simulink model "full_block_trim"  (R2014a)
settings: Solver=ode45  StartTime=0.0  StopTime=500.0  RelTol=1e-3
values from neighbouring files (symbols this model uses):
  alpha_dot = 0    [init_coeff_Cessna.m]
  b = 10.911    [init_coeff_Cessna.m]
  c_bar = 1.493    [init_coeff_Cessna.m]
  c_l_beta = -0.089    [init_coeff_Cessna.m]
  c_l_delta_a = -0.09    [init_coeff_Cessna.m]
  c_l_delta_r = 0.0147    [init_coeff_Cessna.m]
  c_l_p = -0.47    [init_coeff_Cessna.m]
  c_l_r = 0.096    [init_coeff_Cessna.m]
  cd0 = 0.036    [init_coeff_Cessna.m]
  cd_alpha = 0.13    [init_coeff_Cessna.m]
  cd_beta = 0.17    [init_coeff_Cessna.m]
  cd_delta_e = 0.06    [init_coeff_Cessna.m]
  cl0 = 0.25    [init_coeff_Cessna.m]
  cl_alpha = 4.47    [init_coeff_Cessna.m]
  cl_delta_e = 0.3476    [init_coeff_Cessna.m]
  cl_q = 3.9    [init_coeff_Cessna.m]
  cm0 = -0.02    [init_coeff_Cessna.m]
  cm_alpha = -1.8    [init_coeff_Cessna.m]
  cm_alpha_dot = 0.0    (= 0)    [init_coeff_Cessna.m]
  cm_delta_e = -1.28    [init_coeff_Cessna.m]
  cn_beta = 0.065    [init_coeff_Cessna.m]
  cn_delta_a = -0.0053    [init_coeff_Cessna.m]
  cn_delta_r = -0.0657    [init_coeff_Cessna.m]
  cn_p = -0.03    [init_coeff_Cessna.m]
  cn_r = -0.99    [init_coeff_Cessna.m]
  cy_beta = -0.31    [init_coeff_Cessna.m]
  cy_delta_a = 0    [init_coeff_Cessna.m]
  cy_p = -0.037    [init_coeff_Cessna.m]
  cy_r = 0.21    [init_coeff_Cessna.m]
  Ixx = 1285.31    [init_coeff_Cessna.m]
  Ixy = 0.0    (= 0)    [init_coeff_Cessna.m]
  Ixz = 0.0    (= 0)    [init_coeff_Cessna.m]
  Iyx = Ixy    (= 0)    [init_coeff_Cessna.m]
  Iyy = 1824.93    [init_coeff_Cessna.m]
  Iyz = 0.0    (= 0)    [init_coeff_Cessna.m]
  Izx = Ixz    (= 0)    [init_coeff_Cessna.m]
  Izy = Iyz    (= 0)    [init_coeff_Cessna.m]
  Izz = 2666.893    [init_coeff_Cessna.m]
  k_drag = 0.0830304    [init_coeff_Cessna.m]
  p_init = 0    [trim_simulate.m]
  phi_init = 0    [trim_simulate.m]
  psi_init = 0    [trim_simulate.m]
  q_init = 0    [trim_simulate.m]
  r_init = 0    [trim_simulate.m]
  S = 16.1651    [init_coeff_Cessna.m]
  theta_init = 0.0105    [trim_simulate.m]
  u_init = 80.00    (= 80)    [trim_simulate.m]
  v_init = 0.00    (= 0)    [trim_simulate.m]
  W = mass*g    (= 10223.948)    [init_coeff_Cessna.m]
  w_init = 0    [trim_simulate.m]
  xe_init = 0    [trim_simulate.m]
  ye_init = 0    [trim_simulate.m]
  ze_init = -200    [trim_simulate.m]
libraries: aerolibobsolete x1, aerolibatmos2 x1, aerolibtransform2 x1, aerolibasang x1
settings Model: Creator=sajith  LastModifiedBy=sajith
settings DataIOCC: SignalLoggingSaveFormat=ModelDataLogs
settings OptimizationCC: ExpressionDepthLimit=2147483647
settings DebuggingCC: UnderspecifiedInitializationDetection=Classic  FcnCallInpInsideContextMsg=UseLocalSettings  StateNameClashWarn=warning
settings SFSimCC: SimParseCustomCode=off
settings GRTTargetCC: CombineOutputUpdateFcns=off  GRTInterface=on

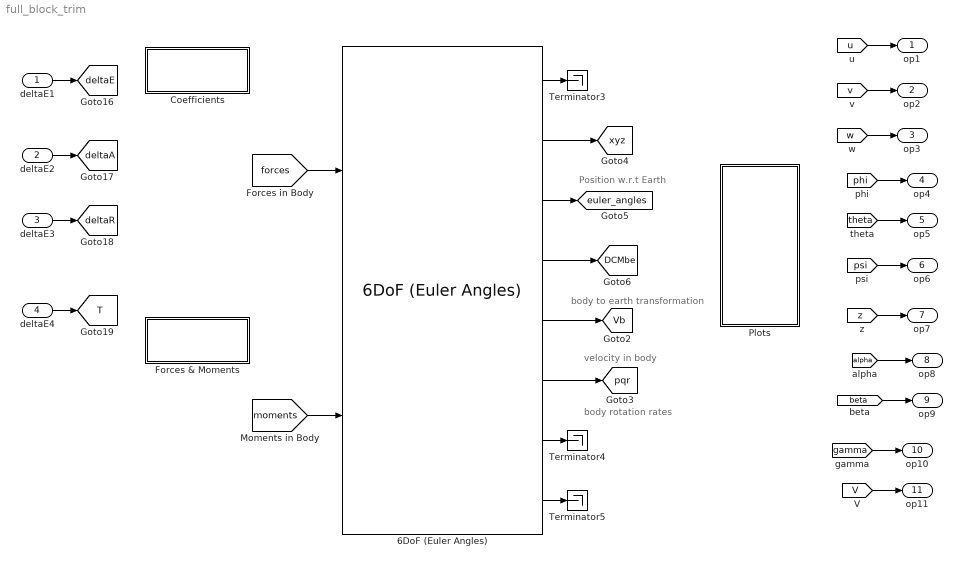
== system full_block_trim ==
  note: velocity in body
  note: body rotation rates
  note: body to earth transformation
  note: Position w.r.t Earth
  deltaE1 : Inport
  deltaE2 : Inport  Port=2
  deltaE3 : Inport  Port=3
  deltaE4 : Inport  Port=4
  6DoF (Euler Angles) : aerolibobsolete/6DoF (Euler Angles)  units=Metric (MKS)  mtype=Fixed  rep=Euler Angles  xme_0=[xe_init ye_init ze_init]  Vm_0=[u_init v_init w_init]  eul_0=[phi_init theta_init psi_init]  pm_0=[p_init q_init r_init]  mass_0=mass  mass_e=0.5  mass_f=2.0  inertia=[Ixx Ixy Ixz;Iyx Iyy Iyz;Izx Izy Izz]  inertia_e=eye(3)  inertia_f=2*eye(3)  k_quat=1.0
  Coefficients : Subsystem
  Forces & Moments : Subsystem
  Plots : Subsystem
  Terminator3 : Terminator
  Terminator4 : Terminator
  Terminator5 : Terminator
  op1 : Outport
  op2 : Outport  Port=2
  op3 : Outport  Port=3
  op4 : Outport  Port=4
  op5 : Outport  Port=5
  op6 : Outport  Port=6
  op7 : Outport  Port=7
  op8 : Outport  Port=8
  op9 : Outport  Port=9
  op10 : Outport  Port=10
  op11 : Outport  Port=11
  tag scope: DCMbe=global, T=global, Vb=global, deltaA=global, deltaE=global, deltaR=global, euler_angles=global, pqr=global, xyz=global
  wires:
  deltaE2/1 -> [deltaA]
  deltaE3/1 -> [deltaR]
  deltaE1/1 -> [deltaE]
  deltaE4/1 -> [T]
  [u] -> op1/1
  [v] -> op2/1
  [w] -> op3/1
  [phi] -> op4/1
  [theta] -> op5/1
  [psi] -> op6/1
  [z] -> op7/1
  [alpha] -> op8/1
  [beta] -> op9/1
  [gamma] -> op10/1
  [V] -> op11/1
  [forces] -> 6DoF (Euler Angles)/1
  [moments] -> 6DoF (Euler Angles)/2
  6DoF (Euler Angles)/2 -> [xyz]
  6DoF (Euler Angles)/3 -> [euler_angles]
  6DoF (Euler Angles)/4 -> [DCMbe]
  6DoF (Euler Angles)/6 -> [pqr]
  6DoF (Euler Angles)/5 -> [Vb]
  6DoF (Euler Angles)/1 -> Terminator3/1
  6DoF (Euler Angles)/7 -> Terminator4/1
  6DoF (Euler Angles)/8 -> Terminator5/1

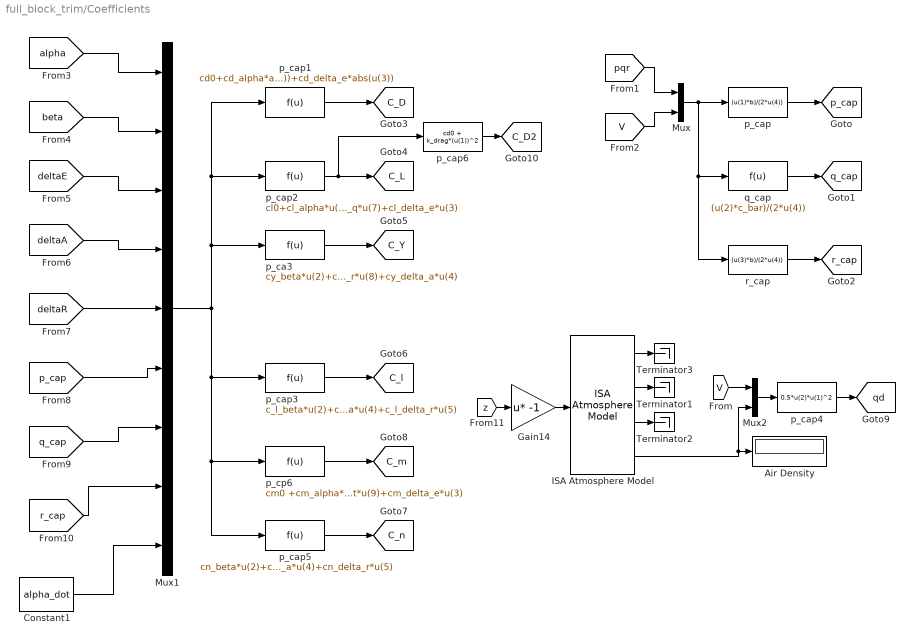
== system full_block_trim/Coefficients ==
  Air Density : Display
  Constant1 : Constant  Value=alpha_dot
  Gain14 : Gain  Gain=-1  Multiplication=Matrix(u*K)
  ISA Atmosphere Model : aerolibatmos2/ISA Atmosphere Model  custom=off  g=9.80665  gamma=1.4  R=287.0531  L=0.0065  h_trop=11000  h_strat=20000  rho0=1.225  P0=101325  T0=288.15  h0=0
  Mux : Mux  Inputs=2
  Mux1 : Mux  Inputs=9
  Mux2 : Mux  Inputs=2
  Terminator1 : Terminator
  Terminator2 : Terminator
  Terminator3 : Terminator
  p_ca3 : Fcn  Expr=cy_beta*u(2)+cy_p*u(6)+cy_r*u(8)+cy_delta_a*u(4)
  p_cap : Fcn  Expr=(u(1)*b)/(2*u(4))
  p_cap1 : Fcn  Expr=cd0+cd_alpha*abs(u(1))+cd_beta*abs(u(2))+cd_delta_e*abs(u(3))
  p_cap2 : Fcn  Expr=cl0+cl_alpha*u(1)+cl_q*u(7)+cl_delta_e*u(3)
  p_cap3 : Fcn  Expr=c_l_beta*u(2)+c_l_p*u(6)+c_l_r*u(8)+c_l_delta_a*u(4)+c_l_delta_r*u(5)
  p_cap4 : Fcn  Expr=0.5*u(2)*u(1)^2
  p_cap5 : Fcn  Expr=cn_beta*u(2)+cn_p*u(6)+cn_r*u(8)+cn_delta_a*u(4)+cn_delta_r*u(5)
  p_cap6 : Fcn  Expr=cd0 + k_drag*(u(1))^2
  p_cp6 : Fcn  Expr=cm0 +cm_alpha*u(1)+cm_alpha_dot*u(9)+cm_delta_e*u(3)
  q_cap : Fcn  Expr=(u(2)*c_bar)/(2*u(4))
  r_cap : Fcn  Expr=(u(3)*b)/(2*u(4))
  tag scope: C_D2=global, C_D=global, C_L=global, C_Y=global, C_l=global, C_m=global, C_n=global, p_cap=global, q_cap=global, qd=global, r_cap=global
  wires:
  [pqr] -> Mux/1
  [V] -> Mux/2
  Mux/1 -> p_cap/1, q_cap/1, r_cap/1
  p_cap/1 -> [p_cap]
  q_cap/1 -> [q_cap]
  r_cap/1 -> [r_cap]
  [alpha] -> Mux1/1
  [beta] -> Mux1/2
  [deltaE] -> Mux1/3
  [deltaA] -> Mux1/4
  [deltaR] -> Mux1/5
  [p_cap] -> Mux1/6
  [q_cap] -> Mux1/7
  [r_cap] -> Mux1/8
  Constant1/1 -> Mux1/9
  Mux1/1 -> p_cap1/1, p_cap2/1, p_ca3/1, p_cap3/1, p_cp6/1, p_cap5/1
  p_cap1/1 -> [C_D]
  p_ca3/1 -> [C_Y]
  p_cap3/1 -> [C_l]
  p_cap5/1 -> [C_n]
  p_cp6/1 -> [C_m]
  [V] -> Mux2/1
  Mux2/1 -> p_cap4/1
  p_cap4/1 -> [qd]
  ISA Atmosphere Model/4 -> Air Density/1, Mux2/2
  Gain14/1 -> ISA Atmosphere Model/1
  [z] -> Gain14/1
  ISA Atmosphere Model/1 -> Terminator3/1
  ISA Atmosphere Model/2 -> Terminator1/1
  ISA Atmosphere Model/3 -> Terminator2/1
  p_cap2/1 -> p_cap6/1, [C_L]
  p_cap6/1 -> [C_D2]

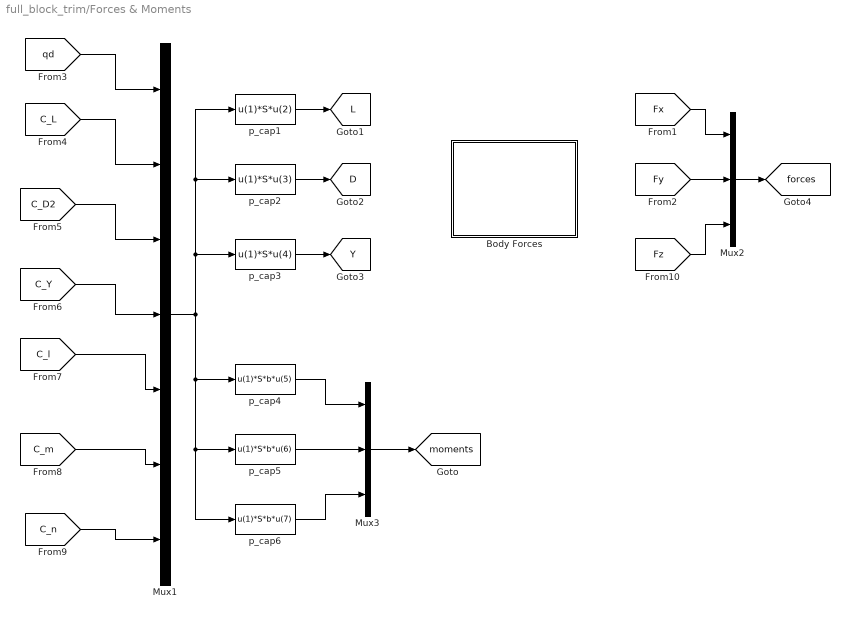
== system full_block_trim/Forces & Moments ==
  Body Forces : Subsystem
  Mux1 : Mux  Inputs=7
  Mux2 : Mux  Inputs=3
  Mux3 : Mux  Inputs=3
  p_cap1 : Fcn  Expr=u(1)*S*u(2)
  p_cap2 : Fcn  Expr=u(1)*S*u(3)
  p_cap3 : Fcn  Expr=u(1)*S*u(4)
  p_cap4 : Fcn  Expr=u(1)*S*b*u(5)
  p_cap5 : Fcn  Expr=u(1)*S*b*u(6)
  p_cap6 : Fcn  Expr=u(1)*S*b*u(7)
  tag scope: D=global, L=global, Y=global, forces=global, moments=global
  wires:
  [qd] -> Mux1/1
  [C_L] -> Mux1/2
  [C_D2] -> Mux1/3
  [C_Y] -> Mux1/4
  [C_l] -> Mux1/5
  [C_m] -> Mux1/6
  [C_n] -> Mux1/7
  Mux1/1 -> p_cap1/1, p_cap2/1, p_cap3/1, p_cap4/1, p_cap5/1, p_cap6/1
  p_cap4/1 -> Mux3/1
  p_cap5/1 -> Mux3/2
  p_cap6/1 -> Mux3/3
  Mux3/1 -> [moments]
  p_cap1/1 -> [L]
  p_cap2/1 -> [D]
  p_cap3/1 -> [Y]
  Mux2/1 -> [forces]
  [Fy] -> Mux2/2
  [Fx] -> Mux2/1
  [Fz] -> Mux2/3

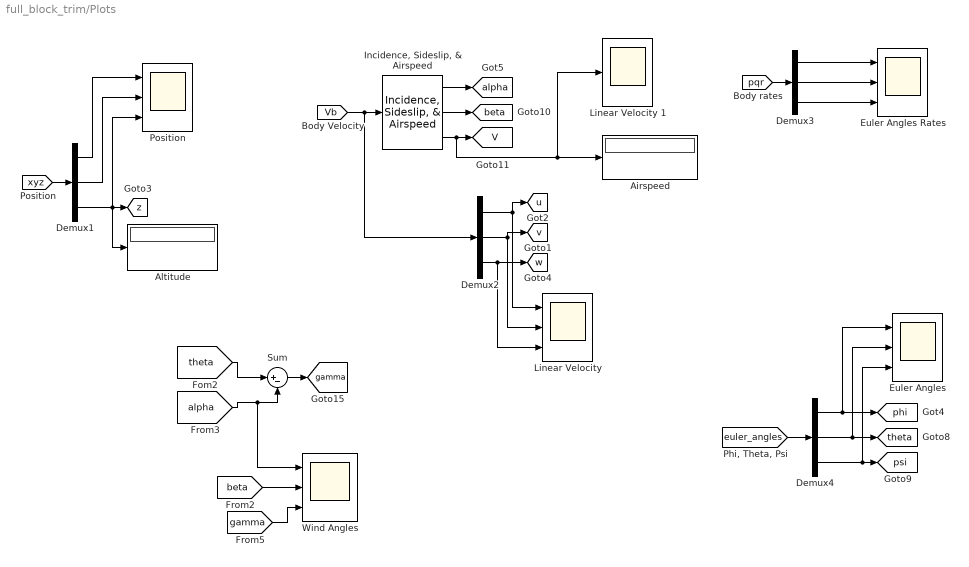
== system full_block_trim/Plots ==
  Airspeed : Display
  Altitude : Display
  Demux{1..4} (4 alike) : Demux  Outputs=3
  Euler Angles : Scope  NumInputPorts=3
      settings: YMin=-5~-5~-5  YMax=5~5~5  SaveName=ScopeData2
  Euler Angles Rates : Scope  NumInputPorts=3
      settings: YMin=-5~-5~-5  YMax=5~5~5  SaveName=ScopeData3
  "Incidence, Sideslip, & Airspeed" : aerolibasang/Incidence, Sideslip, & Airspeed
  "Linear Velocity " : Scope  NumInputPorts=3
      settings: YMin=-5~-5~-5  YMax=5~5~5  SaveName=ScopeData4
  Linear Velocity 1 : Scope
      settings: SaveName=ScopeData5
  Position : Scope  NumInputPorts=3
      settings: YMin=-5~-5~-5  YMax=5~5~5
  Sum : Sum  Inputs=|+-
  Wind Angles : Scope  NumInputPorts=3
      settings: YMin=-5~-5~-5  YMax=5~5~5
  tag scope: V=global, alpha=global, beta=global, gamma=global, phi=global, psi=global, theta=global, u=global, v=global, w=global, z=global
  wires:
  Demux1/1 -> Position/1
  Demux1/2 -> Position/2
  Demux1/3 -> Altitude/1, [z], Position/3
  Demux2/3 -> [w], "Linear Velocity "/3
  Demux2/2 -> [v], "Linear Velocity "/2
  Demux2/1 -> [u], "Linear Velocity "/1
  Demux4/3 -> [psi], Euler Angles/3
  Demux4/2 -> [theta], Euler Angles/2
  Demux4/1 -> [phi], Euler Angles/1
  "Incidence, Sideslip, & Airspeed"/1 -> [alpha]
  "Incidence, Sideslip, & Airspeed"/2 -> [beta]
  "Incidence, Sideslip, & Airspeed"/3 -> [V], Linear Velocity 1/1, Airspeed/1
  [theta] -> Sum/1
  [alpha] -> Sum/2, Wind Angles/1
  Sum/1 -> [gamma]
  [beta] -> Wind Angles/2
  [gamma] -> Wind Angles/3
  [xyz] -> Demux1/1
  [euler_angles] -> Demux4/1
  [Vb] -> Demux2/1, "Incidence, Sideslip, & Airspeed"/1
  [pqr] -> Demux3/1
  Demux3/1 -> Euler Angles Rates/1
  Demux3/2 -> Euler Angles Rates/2
  Demux3/3 -> Euler Angles Rates/3

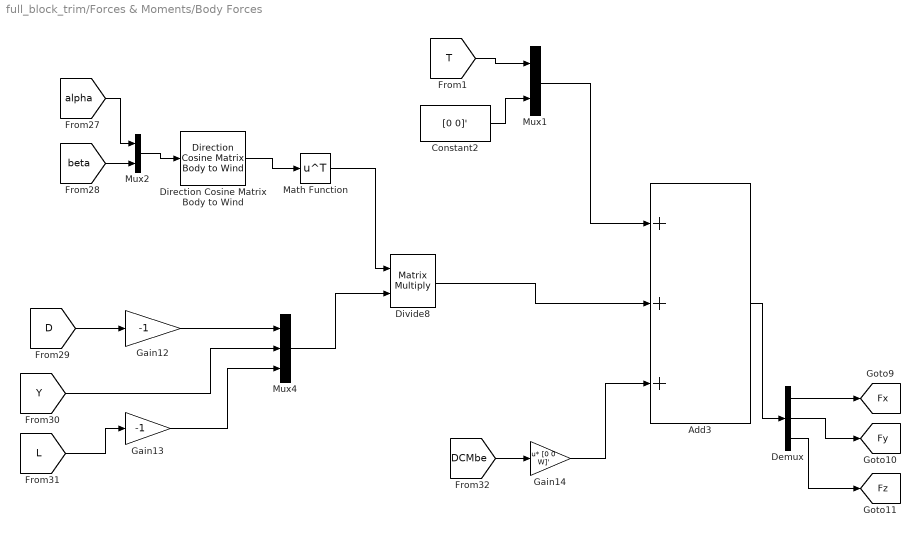
== system full_block_trim/Forces & Moments/Body Forces ==
  Add3 : Sum  Inputs=+++
  Constant2 : Constant  Value=[0 0]'
  Demux : Demux  Outputs=3
  Direction Cosine Matrix Body to Wind : aerolibtransform2/Direction Cosine Matrix Body to Wind
  Divide8 : Product  Inputs=**  Multiplication=Matrix(*)
  Gain12 : Gain  Gain=-1
  Gain13 : Gain  Gain=-1
  Gain14 : Gain  Gain=[0 0 W]'  Multiplication=Matrix(u*K)
  Math Function : Math  Operator=transpose  SaturateOnIntegerOverflow=on
  Mux1 : Mux  Inputs=2
  Mux2 : Mux  Inputs=2
  Mux4 : Mux  Inputs=3
  tag scope: Fx=global, Fy=global, Fz=global
  wires:
  Direction Cosine Matrix Body to Wind/1 -> Math Function/1
  [alpha] -> Mux2/1
  [beta] -> Mux2/2
  Mux2/1 -> Direction Cosine Matrix Body to Wind/1
  Math Function/1 -> Divide8/1
  [D] -> Gain12/1
  [L] -> Gain13/1
  Gain12/1 -> Mux4/1
  [Y] -> Mux4/2
  Gain13/1 -> Mux4/3
  [DCMbe] -> Gain14/1
  Add3/1 -> Demux/1
  Demux/1 -> [Fx]
  Demux/2 -> [Fy]
  Demux/3 -> [Fz]
  Gain14/1 -> Add3/3
  Mux4/1 -> Divide8/2
  [T] -> Mux1/1
  Constant2/1 -> Mux1/2
  Mux1/1 -> Add3/1
  Divide8/1 -> Add3/2
